simulink library "Collector_Unglazed_CONF"  (R2013b)
settings: Solver=ode45  StartTime=0.0  StopTime=10.0  RelTol=1e-3
libraries: carnot x2
settings Model: Creator=lena.frank  LastModifiedBy=drhf

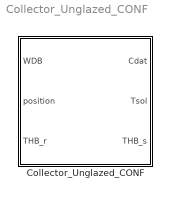
== system Collector_Unglazed_CONF ==
  Collector_Unglazed_CONF : Subsystem  mask(configurated Solar Thermal Collector){parameterfile=DefaultCollectorUnglazed, tini=20, Ncollector=1}
      mask prompts: parameterfile "Parameter set"; tini "Inital temperature in °C"; Ncollector "Number of collectors in parallel"
      mask help:
      | Dynamic 1-node collector model according to EN 12975 standard.
      | This block uses predefined parameter sets.
      mask init:
      | % path definitions
      | intpath = fullfile(path_carnot('intlibsl'), 'Source','Solar_Thermal', ...
      |     'Collector_Unglazed_CONF','parameter_set');
      | pubpath = fullfile(path_carnot('libsl'), 'Source','Solar_Thermal', ...
      |     'Collector_Unglazed_CONF','parameter_set');
      | 
      | [namelist, lib] = CarnotCallbacks_getConfNamelist(intpath,pubpath);
      | 
      | % set namelist in mask
      | if ~lib
      |     myMaskStylesVar{1} = ['popup(', namelist,')'];
      |     myMaskStylesVar{2} = 'edit';
      |     myMaskStylesVar{3} = 'edit';
      |     set_param(gcb, 'MaskStyles', myMaskStylesVar);
      | end
      | 
      | if exist(fullfile(intpath,[parameterfile '.mat']))
      |     load(fullfile(intpath,parameterfile));
      | else
      |     load(fullfile(pubpath,parameterfile));
      | end
      mask Help: web(fullfile(path_carnot('help'),'Collector_Unglazed.html'),'-helpbrowser')
      mask TypeOptions parameterfile: DefaultCollectorUnglazed | NotYet_Isocal_Absorber
      mask Display:
      | % user defined picture file
      | picfile = fullfile(path_carnot('intlibsl'), ...
      |     'Source','Solar_Thermal','Collector_Unglazed_CONF','parameter_set', ...
      |      'Collector_CONF.jpg');
      | 
      | pic = false;
      | 
      | % show internal picture if defined
      | if ~BlockIsInCarnotLibrary    % if not located in library any more
      |     if exist(picfile)
      |         image(imread(picfile), [0, 0, 1, 1])
      |         set_param(gcb, 'BackgroundColor', 'White')
      |         pic = true;
      |     end
      | end
      | 
      | if ~pic % show public picture
      |     plot([0,70,70,0,0]/100,[-0,-0,5,5,-0]/100,[30,30,100,100,30]/100,...
      |         [100,94,94,100,100]/100,[32,1]/100,[94,5]/100,[40,10]/100,...
      |         [94,5]/100,[49,19]/100,[94,5]/100,[57,27]/100,[94,5]/100,[65,35]/100,...
      |         [94,5]/100,[73,43]/100,[94,5]/100,[82,51]/100,[94,5]/100,[90,60]/100,...
      |         [94,5]/100,[98,68]/100,[94,5]/100)
      |     set_param(gcb, 'BackgroundColor', 'Yellow')
      | end
      | 
      | % Show port labels: same as port labels in the subsystem,
      | % but display with a picture covers the text. Have to reprint it.
      | port_label('input',1,'WDB')
      | port_label('input',2,'position')
      | port_label('input',3,'THB_r')
      | port_label('output',1,'Cdat')
      | port_label('output',2,'Tsol')
      | port_label('output',3,'THB_s')

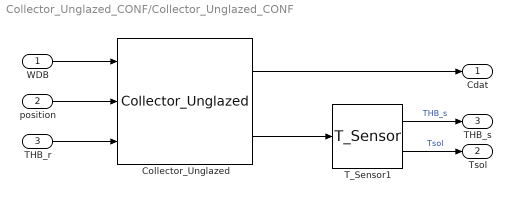
== system Collector_Unglazed_CONF/Collector_Unglazed_CONF ==
  WDB : Inport
  position : Inport  Port=2
  THB_r : Inport  Port=3
  Collector_Unglazed : carnot/Source/Solar_Thermal/Collector_Unglazed  acol=USTC.Acoll  len=USTC.len  fta=USTC.fta  e_sky=USTC.eps  uc0=USTC.u0c  uc1=USTC.u1c  uc0loss=USTC.u0l  uc1loss=USTC.u1l  uc0gain=USTC.u0g  uc1gain=USTC.u1g  uc1eta0=USTC.u1e  hi=USTC.hi  c_abs=USTC.capa  c_fl=USTC.capf  lin=USTC.lin  qua=USTC.qua  tini=tini  nodes=USTC.nodes
  T_Sensor1 : carnot/Control/T_Sensor  tc=USTC.SensorTimeConstant  t0=tini
  Cdat : Outport
  Tsol : Outport  Port=2
  THB_s : Outport  Port=3
  wires:
  T_Sensor1/2 -> Tsol/1  "Tsol"
  T_Sensor1/1 -> THB_s/1  "THB_s"
  Collector_Unglazed/2 -> T_Sensor1/1
  WDB/1 -> Collector_Unglazed/1
  position/1 -> Collector_Unglazed/2
  THB_r/1 -> Collector_Unglazed/3
  Collector_Unglazed/1 -> Cdat/1
